simulink model "simulation"  (R2023b)
settings: Solver=VariableStepAuto  StartTime=0.0  StopTime=T  RelTol=1e-3
values from neighbouring files (symbols this model uses):
  A = [U'*inv(M)' ... (first row only)    [getTau.m]    (also in init.m = [zeros(numRoots+1), eye(numRoots+1))
  B = M \ K    [getTau.m]    (also in init.m = [zeros(numRoots+1,1); M^-1*U])
  C = subs(C, [om1 om2 om3], omega)    [getTau.m]    (also in init.m = eye(numRoots*2+2))
  D = zeros((N+1)/2)    [getTrajectory.m]    (also in init.m = zeros(numRoots*2+2, 1))
  Kd = 0    [init.m]
  Kp = 0    [init.m]
  numRoots = 3    [init.m]
  phiL = phiX(:, end)    [init.m]
  phiL_prime = phiX_prime(:,end)    [init.m]
  sampleTime = T/500    (= 0.002)    [init.m]
  tauLim = 100000    [init.m]
  x0 = [0 0 0 0 0 0 0 0]'    [init.m]
settings Model: Creator=cyber_m  LastModifiedBy=cyber_m

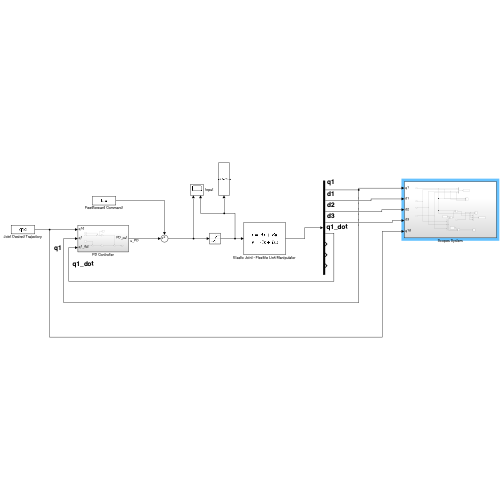
[thumbnail: Simulink's stored preview of the top-level diagram]
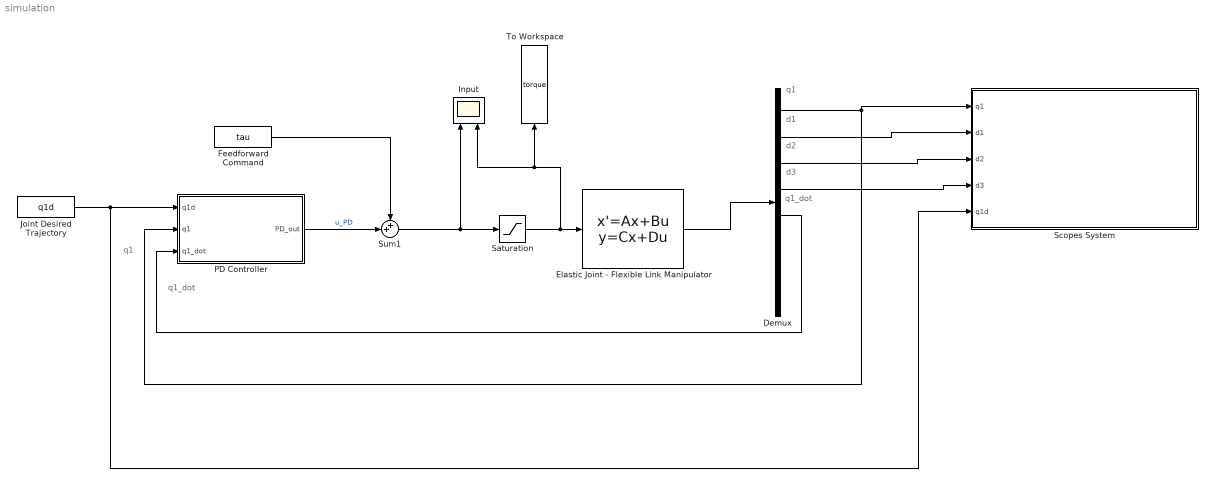
== system simulation ==
  note: q1
  note: d1
  note: d2
  note: d3
  note: q1_dot
  note: q1_dot
  note: q1
  Demux : Demux  Outputs=numRoots*2+2
  Elastic Joint - Flexible Link Manipulator : StateSpace  A=A  B=B  C=C  D=D  InitialCondition=x0
  Feedforward Command : FromWorkspace  VariableName=tau  SampleTime=-1  OutputAfterFinalValue=Setting to zero
  Input : Scope  NumInputPorts=2
  Joint Desired Trajectory : FromWorkspace  VariableName=q1d  SampleTime=-1
  PD Controller : Subsystem
  Saturation : Saturate  UpperLimit=tauLim  LowerLimit=-tauLim
  Scopes System : Subsystem
  Sum1 : Sum  Inputs=++|
  To Workspace : ToWorkspace  VariableName=torque  SampleTime=sampleTime
  wires:
  Elastic Joint - Flexible Link Manipulator/1 -> Demux/1
  Demux/1 -> PD Controller/2(q1), Scopes System/1(q1)
  Demux/2 -> Scopes System/2(d1)
  Demux/3 -> Scopes System/3(d2)
  Demux/4 -> Scopes System/4(d3)
  Saturation/1 -> Elastic Joint - Flexible Link Manipulator/1, Input/2, To Workspace/1
  Feedforward Command/1 -> Sum1/1
  Demux/5 -> PD Controller/3(q1_dot)
  PD Controller/1(PD_out) -> Sum1/2  "u_PD"
  Sum1/1 -> Saturation/1, Input/1
  Joint Desired Trajectory/1 -> PD Controller/1(q1d), Scopes System/5(q1d)

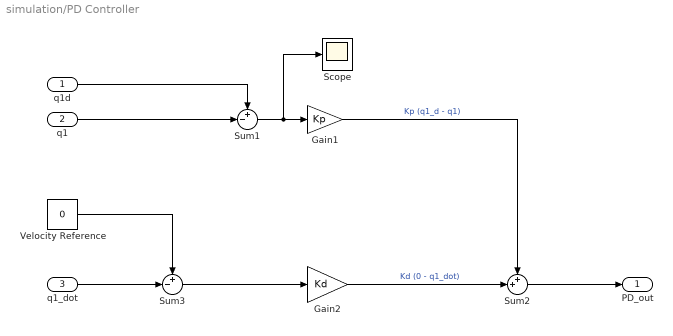
== system simulation/PD Controller ==
  q1d : Inport
  q1 : Inport  Port=2
  q1_dot : Inport  Port=3
  Gain1 : Gain  Gain=Kp
  Gain2 : Gain  Gain=Kd
  Scope : Scope
  Sum1 : Sum  Inputs=+-|
  Sum2 : Sum  Inputs=++|
  Sum3 : Sum  Inputs=+-|
  Velocity Reference : Constant  Value=0
  PD_out : Outport
  wires:
  Sum3/1 -> Gain2/1
  Sum1/1 -> Scope/1, Gain1/1
  Gain1/1 -> Sum2/1  "Kp (q1_d - q1)"
  q1d/1 -> Sum1/1
  q1/1 -> Sum1/2
  q1_dot/1 -> Sum3/2
  Gain2/1 -> Sum2/2  "Kd (0 - q1_dot)"
  Sum2/1 -> PD_out/1
  Velocity Reference/1 -> Sum3/1

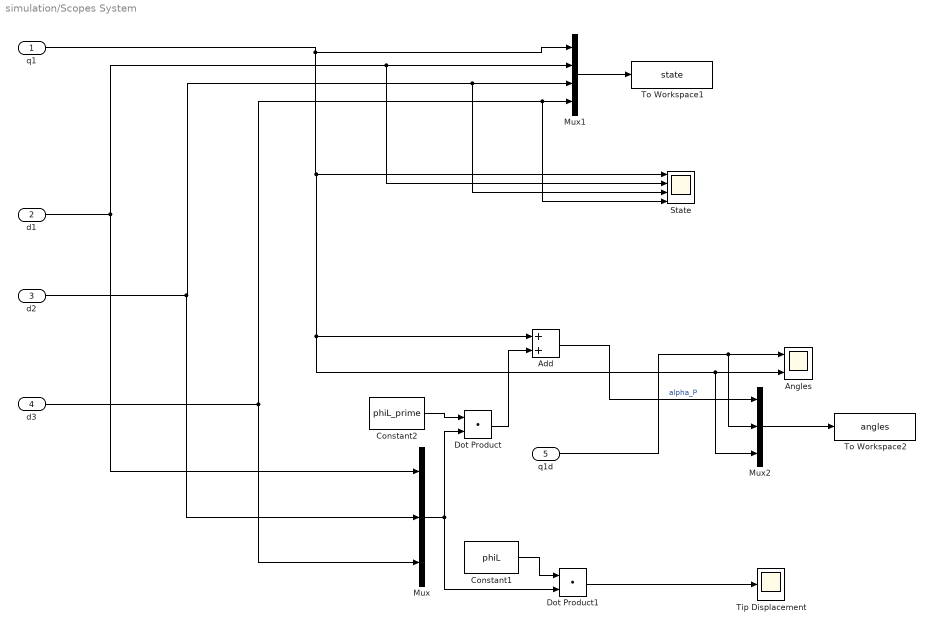
== system simulation/Scopes System ==
  q1 : Inport
  d1 : Inport  Port=2
  d2 : Inport  Port=3
  d3 : Inport  Port=4
  q1d : Inport  Port=5
  Add : Sum
  Angles : Scope  NumInputPorts=2
  Constant1 : Constant  Value=phiL
  Constant2 : Constant  Value=phiL_prime
  Dot Product : DotProduct  OutDataTypeStr=Inherit: Inherit via internal rule
  Dot Product1 : DotProduct  OutDataTypeStr=Inherit: Inherit via internal rule
  Mux : Mux  Inputs=numRoots
  Mux1 : Mux  Inputs=numRoots+1
  Mux2 : Mux  Inputs=numRoots
  State : Scope  NumInputPorts=4
  Tip Displacement : Scope
  To Workspace1 : ToWorkspace  VariableName=state  SampleTime=sampleTime
  To Workspace2 : ToWorkspace  VariableName=angles  SampleTime=sampleTime
  wires:
  Mux/1 -> Dot Product1/2, Dot Product/2
  Dot Product/1 -> Add/2
  Constant2/1 -> Dot Product/1
  d1/1 -> Mux/1, State/2, Mux1/2
  d2/1 -> Mux/2, State/3, Mux1/3
  d3/1 -> Mux/3, Mux1/4, State/4
  q1d/1 -> Mux2/2, Angles/1
  Constant1/1 -> Dot Product1/1
  Dot Product1/1 -> Tip Displacement/1
  Mux2/1 -> To Workspace2/1
  q1/1 -> Mux2/3, Angles/2, Add/1, State/1, Mux1/1
  Mux1/1 -> To Workspace1/1
  Add/1 -> Mux2/1  "alpha_P"
